simulink model "xEMU_SimulationModel3_rule1"  (R2017b)
settings: Solver=ode4  StartTime=0.0  StopTime=8192  FixedStep=0.01  RelTol=1e-3
undefined symbols (not defined in the file): a1, a2, a3, a4, ACO, BAT, Battery, DCT, DRT, EMS, ENV, Fahrzyklus_VS_modell, height_BAT, leistung, lib_bat, Maximum, Maximum_position, Num_cells, P_FC_max_long, P_FC_min_long, P_FC_step_max, Pbat_charge_max, Pbat_discharge_max, Pfc_max, Pfc_min, SOC_tar, time_peaks, TRM, velocity_peaks
libraries: simulink x5
(part 11 of 15)

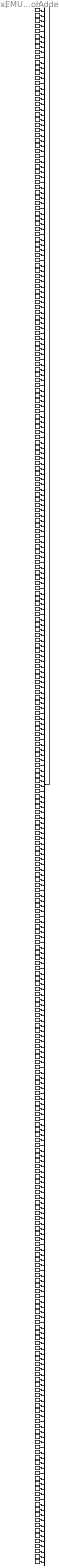
== system xEMU_SimulationModel3_rule1/Battery (BAT)_komplex/Subsystem/Thermal/Coolings/CoolAdder ==
  P_cool : Inport
  Add_FV_{1..300} (300 alike) : Sum  Inputs=-
  Demux : Demux  Outputs=2
  Mux : Mux  Inputs=300
  P_FV : Outport
  wires:
  P_cool/1 -> Demux/1
  Mux/1 -> P_FV/1
  Add_FV_1/1 -> Mux/1
  Add_FV_2/1 -> Mux/2
  Add_FV_3/1 -> Mux/3
  Add_FV_4/1 -> Mux/4
  Add_FV_5/1 -> Mux/5
  Add_FV_6/1 -> Mux/6
  Add_FV_7/1 -> Mux/7
  Add_FV_8/1 -> Mux/8
  Add_FV_9/1 -> Mux/9
  Add_FV_10/1 -> Mux/10
  Add_FV_11/1 -> Mux/11
  Add_FV_12/1 -> Mux/12
  Add_FV_13/1 -> Mux/13
  Add_FV_14/1 -> Mux/14
  Add_FV_15/1 -> Mux/15
  Add_FV_16/1 -> Mux/16
  Add_FV_17/1 -> Mux/17
  Add_FV_18/1 -> Mux/18
  Add_FV_19/1 -> Mux/19
  Add_FV_20/1 -> Mux/20
  Add_FV_21/1 -> Mux/21
  Add_FV_22/1 -> Mux/22
  Add_FV_23/1 -> Mux/23
  Add_FV_24/1 -> Mux/24
  Add_FV_25/1 -> Mux/25
  Add_FV_26/1 -> Mux/26
  Add_FV_27/1 -> Mux/27
  Add_FV_28/1 -> Mux/28
  Add_FV_29/1 -> Mux/29
  Add_FV_30/1 -> Mux/30
  Add_FV_31/1 -> Mux/31
  Add_FV_32/1 -> Mux/32
  Add_FV_33/1 -> Mux/33
  Add_FV_34/1 -> Mux/34
  Add_FV_35/1 -> Mux/35
  Add_FV_36/1 -> Mux/36
  Add_FV_37/1 -> Mux/37
  Add_FV_38/1 -> Mux/38
  Add_FV_39/1 -> Mux/39
  Add_FV_40/1 -> Mux/40
  Add_FV_41/1 -> Mux/41
  Add_FV_42/1 -> Mux/42
  Add_FV_43/1 -> Mux/43
  Add_FV_44/1 -> Mux/44
  Add_FV_45/1 -> Mux/45
  Add_FV_46/1 -> Mux/46
  Add_FV_47/1 -> Mux/47
  Add_FV_48/1 -> Mux/48
  Add_FV_49/1 -> Mux/49
  Add_FV_50/1 -> Mux/50
  Add_FV_51/1 -> Mux/51
  Add_FV_52/1 -> Mux/52
  Add_FV_53/1 -> Mux/53
  Add_FV_54/1 -> Mux/54
  Add_FV_55/1 -> Mux/55
  Add_FV_56/1 -> Mux/56
  Add_FV_57/1 -> Mux/57
  Add_FV_58/1 -> Mux/58
  Add_FV_59/1 -> Mux/59
  Add_FV_60/1 -> Mux/60
  Add_FV_61/1 -> Mux/61
  Add_FV_62/1 -> Mux/62
  Add_FV_63/1 -> Mux/63
  Add_FV_64/1 -> Mux/64
  Add_FV_65/1 -> Mux/65
  Add_FV_66/1 -> Mux/66
  Add_FV_67/1 -> Mux/67
  Add_FV_68/1 -> Mux/68
  Add_FV_69/1 -> Mux/69
  Add_FV_70/1 -> Mux/70
  Add_FV_71/1 -> Mux/71
  Add_FV_72/1 -> Mux/72
  Add_FV_73/1 -> Mux/73
  Add_FV_74/1 -> Mux/74
  Add_FV_75/1 -> Mux/75
  Add_FV_76/1 -> Mux/76
  Add_FV_77/1 -> Mux/77
  Add_FV_78/1 -> Mux/78
  Add_FV_79/1 -> Mux/79
  Add_FV_80/1 -> Mux/80
  Add_FV_81/1 -> Mux/81
  Add_FV_82/1 -> Mux/82
  Add_FV_83/1 -> Mux/83
  Add_FV_84/1 -> Mux/84
  Add_FV_85/1 -> Mux/85
  Add_FV_86/1 -> Mux/86
  Add_FV_87/1 -> Mux/87
  Add_FV_88/1 -> Mux/88
  Add_FV_89/1 -> Mux/89
  Add_FV_90/1 -> Mux/90
  Add_FV_91/1 -> Mux/91
  Add_FV_92/1 -> Mux/92
  Add_FV_93/1 -> Mux/93
  Add_FV_94/1 -> Mux/94
  Add_FV_95/1 -> Mux/95
  Add_FV_96/1 -> Mux/96
  Add_FV_97/1 -> Mux/97
  Add_FV_98/1 -> Mux/98
  Add_FV_99/1 -> Mux/99
  Add_FV_100/1 -> Mux/100
  Add_FV_101/1 -> Mux/101
  Add_FV_102/1 -> Mux/102
  Add_FV_103/1 -> Mux/103
  Add_FV_104/1 -> Mux/104
  Add_FV_105/1 -> Mux/105
  Add_FV_106/1 -> Mux/106
  Add_FV_107/1 -> Mux/107
  Add_FV_108/1 -> Mux/108
  Add_FV_109/1 -> Mux/109
  Add_FV_110/1 -> Mux/110
  Add_FV_111/1 -> Mux/111
  Add_FV_112/1 -> Mux/112
  Add_FV_113/1 -> Mux/113
  Add_FV_114/1 -> Mux/114
  Add_FV_115/1 -> Mux/115
  Add_FV_116/1 -> Mux/116
  Add_FV_117/1 -> Mux/117
  Add_FV_118/1 -> Mux/118
  Add_FV_119/1 -> Mux/119
  Add_FV_120/1 -> Mux/120
  Add_FV_121/1 -> Mux/121
  Add_FV_122/1 -> Mux/122
  Add_FV_123/1 -> Mux/123
  Add_FV_124/1 -> Mux/124
  Add_FV_125/1 -> Mux/125
  Add_FV_126/1 -> Mux/126
  Add_FV_127/1 -> Mux/127
  Add_FV_128/1 -> Mux/128
  Add_FV_129/1 -> Mux/129
  Add_FV_130/1 -> Mux/130
  Add_FV_131/1 -> Mux/131
  Add_FV_132/1 -> Mux/132
  Add_FV_133/1 -> Mux/133
  Add_FV_134/1 -> Mux/134
  Add_FV_135/1 -> Mux/135
  Add_FV_136/1 -> Mux/136
  Add_FV_137/1 -> Mux/137
  Add_FV_138/1 -> Mux/138
  Add_FV_139/1 -> Mux/139
  Add_FV_140/1 -> Mux/140
  Add_FV_141/1 -> Mux/141
  Add_FV_142/1 -> Mux/142
  Add_FV_143/1 -> Mux/143
  Add_FV_144/1 -> Mux/144
  Add_FV_145/1 -> Mux/145
  Add_FV_146/1 -> Mux/146
  Add_FV_147/1 -> Mux/147
  Add_FV_148/1 -> Mux/148
  Add_FV_149/1 -> Mux/149
  Add_FV_150/1 -> Mux/150
  Add_FV_151/1 -> Mux/151
  Add_FV_152/1 -> Mux/152
  Add_FV_153/1 -> Mux/153
  Add_FV_154/1 -> Mux/154
  Add_FV_155/1 -> Mux/155
  Add_FV_156/1 -> Mux/156
  Add_FV_157/1 -> Mux/157
  Add_FV_158/1 -> Mux/158
  Add_FV_159/1 -> Mux/159
  Add_FV_160/1 -> Mux/160
  Add_FV_161/1 -> Mux/161
  Add_FV_162/1 -> Mux/162
  Add_FV_163/1 -> Mux/163
  Add_FV_164/1 -> Mux/164
  Add_FV_165/1 -> Mux/165
  Add_FV_166/1 -> Mux/166
  Add_FV_167/1 -> Mux/167
  Add_FV_168/1 -> Mux/168
  Add_FV_169/1 -> Mux/169
  Add_FV_170/1 -> Mux/170
  Add_FV_171/1 -> Mux/171
  Add_FV_172/1 -> Mux/172
  Add_FV_173/1 -> Mux/173
  Add_FV_174/1 -> Mux/174
  Add_FV_175/1 -> Mux/175
  Add_FV_176/1 -> Mux/176
  Add_FV_177/1 -> Mux/177
  Add_FV_178/1 -> Mux/178
  Add_FV_179/1 -> Mux/179
  Add_FV_180/1 -> Mux/180
  Add_FV_181/1 -> Mux/181
  Add_FV_182/1 -> Mux/182
  Add_FV_183/1 -> Mux/183
  Add_FV_184/1 -> Mux/184
  Add_FV_185/1 -> Mux/185
  Add_FV_186/1 -> Mux/186
  Add_FV_187/1 -> Mux/187
  Add_FV_188/1 -> Mux/188
  Add_FV_189/1 -> Mux/189
  Add_FV_190/1 -> Mux/190
  Add_FV_191/1 -> Mux/191
  Add_FV_192/1 -> Mux/192
  Add_FV_193/1 -> Mux/193
  Add_FV_194/1 -> Mux/194
  Add_FV_195/1 -> Mux/195
  Add_FV_196/1 -> Mux/196
  Add_FV_197/1 -> Mux/197
  Add_FV_198/1 -> Mux/198
  Add_FV_199/1 -> Mux/199
  Add_FV_200/1 -> Mux/200
  Add_FV_201/1 -> Mux/201
  Add_FV_202/1 -> Mux/202
  Add_FV_203/1 -> Mux/203
  Add_FV_204/1 -> Mux/204
  Add_FV_205/1 -> Mux/205
  Add_FV_206/1 -> Mux/206
  Add_FV_207/1 -> Mux/207
  Add_FV_208/1 -> Mux/208
  Add_FV_209/1 -> Mux/209
  Add_FV_210/1 -> Mux/210
  Add_FV_211/1 -> Mux/211
  Add_FV_212/1 -> Mux/212
  Add_FV_213/1 -> Mux/213
  Add_FV_214/1 -> Mux/214
  Add_FV_215/1 -> Mux/215
  Add_FV_216/1 -> Mux/216
  Add_FV_217/1 -> Mux/217
  Add_FV_218/1 -> Mux/218
  Add_FV_219/1 -> Mux/219
  Add_FV_220/1 -> Mux/220
  Add_FV_221/1 -> Mux/221
  Add_FV_222/1 -> Mux/222
  Add_FV_223/1 -> Mux/223
  Add_FV_224/1 -> Mux/224
  Add_FV_225/1 -> Mux/225
  Add_FV_226/1 -> Mux/226
  Add_FV_227/1 -> Mux/227
  Add_FV_228/1 -> Mux/228
  Add_FV_229/1 -> Mux/229
  Add_FV_230/1 -> Mux/230
  Add_FV_231/1 -> Mux/231
  Add_FV_232/1 -> Mux/232
  Add_FV_233/1 -> Mux/233
  Add_FV_234/1 -> Mux/234
  Add_FV_235/1 -> Mux/235
  Add_FV_236/1 -> Mux/236
  Add_FV_237/1 -> Mux/237
  Add_FV_238/1 -> Mux/238
  Add_FV_239/1 -> Mux/239
  Add_FV_240/1 -> Mux/240
  Add_FV_241/1 -> Mux/241
  Add_FV_242/1 -> Mux/242
  Add_FV_243/1 -> Mux/243
  Add_FV_244/1 -> Mux/244
  Add_FV_245/1 -> Mux/245
  Add_FV_246/1 -> Mux/246
  Add_FV_247/1 -> Mux/247
  Add_FV_248/1 -> Mux/248
  Add_FV_249/1 -> Mux/249
  Add_FV_250/1 -> Mux/250
  Add_FV_251/1 -> Mux/251
  Add_FV_252/1 -> Mux/252
  Add_FV_253/1 -> Mux/253
  Add_FV_254/1 -> Mux/254
  Add_FV_255/1 -> Mux/255
  Add_FV_256/1 -> Mux/256
  Add_FV_257/1 -> Mux/257
  Add_FV_258/1 -> Mux/258
  Add_FV_259/1 -> Mux/259
  Add_FV_260/1 -> Mux/260
  Add_FV_261/1 -> Mux/261
  Add_FV_262/1 -> Mux/262
  Add_FV_263/1 -> Mux/263
  Add_FV_264/1 -> Mux/264
  Add_FV_265/1 -> Mux/265
  Add_FV_266/1 -> Mux/266
  Add_FV_267/1 -> Mux/267
  Add_FV_268/1 -> Mux/268
  Add_FV_269/1 -> Mux/269
  Add_FV_270/1 -> Mux/270
  Add_FV_271/1 -> Mux/271
  Add_FV_272/1 -> Mux/272
  Add_FV_273/1 -> Mux/273
  Add_FV_274/1 -> Mux/274
  Add_FV_275/1 -> Mux/275
  Add_FV_276/1 -> Mux/276
  Add_FV_277/1 -> Mux/277
  Add_FV_278/1 -> Mux/278
  Add_FV_279/1 -> Mux/279
  Add_FV_280/1 -> Mux/280
  Add_FV_281/1 -> Mux/281
  Add_FV_282/1 -> Mux/282
  Add_FV_283/1 -> Mux/283
  Add_FV_284/1 -> Mux/284
  Add_FV_285/1 -> Mux/285
  Add_FV_286/1 -> Mux/286
  Add_FV_287/1 -> Mux/287
  Add_FV_288/1 -> Mux/288
  Add_FV_289/1 -> Mux/289
  Add_FV_290/1 -> Mux/290
  Add_FV_291/1 -> Mux/291
  Add_FV_292/1 -> Mux/292
  Add_FV_293/1 -> Mux/293
  Add_FV_294/1 -> Mux/294
  Add_FV_295/1 -> Mux/295
  Add_FV_296/1 -> Mux/296
  Add_FV_297/1 -> Mux/297
  Add_FV_298/1 -> Mux/298
  Add_FV_299/1 -> Mux/299
  Add_FV_300/1 -> Mux/300

== system xEMU_SimulationModel3_rule1/Battery (BAT)_mittel/Battery/ElectricalCircuit/SerialTwoPort_Elem1/Cellelement_Elem1 ==
  OhmicResistance_Elem4 : Subsystem
  ParallelRC_Elem1 : Subsystem
  ParallelRC_Elem2 : Subsystem
  ParallelRC_Elem3 : Subsystem
  SoC : Integrator  InitialCondition=SOC_tar*100  LimitOutput=on  UpperSaturationLimit=100  LowerSaturationLimit=0
  SoCFactor : Gain  Gain=0.0012077
  VoltageSource_Elem5 : Subsystem
  tag scope: SoC1=scoped
  wires:
  [I_CellElement1] -> SoCFactor/1
  SoCFactor/1 -> SoC/1
  SoC/1 -> OhmicResistance_Elem4/2(SoC), VoltageSource_Elem5/2(SoC), ParallelRC_Elem3/2(SoC), ParallelRC_Elem2/2(SoC), ParallelRC_Elem1/2(SoC), [SoC1]
  [T_CellElement1] -> OhmicResistance_Elem4/1(T), VoltageSource_Elem5/1(T), ParallelRC_Elem3/1(T), ParallelRC_Elem2/1(T), ParallelRC_Elem1/1(T)

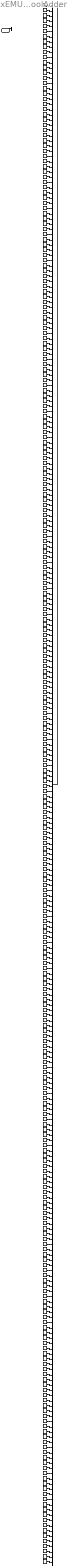
== system xEMU_SimulationModel3_rule1/Battery (BAT)_mittel/Battery/Thermal/Coolings/CoolAdder ==
  P_cool : Inport
  Add_FV_{1..300} (300 alike) : Sum  Inputs=-
  Demux : Demux  Outputs=2
  Mux : Mux  Inputs=300
  P_FV : Outport
  wires:
  P_cool/1 -> Demux/1
  Mux/1 -> P_FV/1
  Add_FV_1/1 -> Mux/1
  Add_FV_2/1 -> Mux/2
  Add_FV_3/1 -> Mux/3
  Add_FV_4/1 -> Mux/4
  Add_FV_5/1 -> Mux/5
  Add_FV_6/1 -> Mux/6
  Add_FV_7/1 -> Mux/7
  Add_FV_8/1 -> Mux/8
  Add_FV_9/1 -> Mux/9
  Add_FV_10/1 -> Mux/10
  Add_FV_11/1 -> Mux/11
  Add_FV_12/1 -> Mux/12
  Add_FV_13/1 -> Mux/13
  Add_FV_14/1 -> Mux/14
  Add_FV_15/1 -> Mux/15
  Add_FV_16/1 -> Mux/16
  Add_FV_17/1 -> Mux/17
  Add_FV_18/1 -> Mux/18
  Add_FV_19/1 -> Mux/19
  Add_FV_20/1 -> Mux/20
  Add_FV_21/1 -> Mux/21
  Add_FV_22/1 -> Mux/22
  Add_FV_23/1 -> Mux/23
  Add_FV_24/1 -> Mux/24
  Add_FV_25/1 -> Mux/25
  Add_FV_26/1 -> Mux/26
  Add_FV_27/1 -> Mux/27
  Add_FV_28/1 -> Mux/28
  Add_FV_29/1 -> Mux/29
  Add_FV_30/1 -> Mux/30
  Add_FV_31/1 -> Mux/31
  Add_FV_32/1 -> Mux/32
  Add_FV_33/1 -> Mux/33
  Add_FV_34/1 -> Mux/34
  Add_FV_35/1 -> Mux/35
  Add_FV_36/1 -> Mux/36
  Add_FV_37/1 -> Mux/37
  Add_FV_38/1 -> Mux/38
  Add_FV_39/1 -> Mux/39
  Add_FV_40/1 -> Mux/40
  Add_FV_41/1 -> Mux/41
  Add_FV_42/1 -> Mux/42
  Add_FV_43/1 -> Mux/43
  Add_FV_44/1 -> Mux/44
  Add_FV_45/1 -> Mux/45
  Add_FV_46/1 -> Mux/46
  Add_FV_47/1 -> Mux/47
  Add_FV_48/1 -> Mux/48
  Add_FV_49/1 -> Mux/49
  Add_FV_50/1 -> Mux/50
  Add_FV_51/1 -> Mux/51
  Add_FV_52/1 -> Mux/52
  Add_FV_53/1 -> Mux/53
  Add_FV_54/1 -> Mux/54
  Add_FV_55/1 -> Mux/55
  Add_FV_56/1 -> Mux/56
  Add_FV_57/1 -> Mux/57
  Add_FV_58/1 -> Mux/58
  Add_FV_59/1 -> Mux/59
  Add_FV_60/1 -> Mux/60
  Add_FV_61/1 -> Mux/61
  Add_FV_62/1 -> Mux/62
  Add_FV_63/1 -> Mux/63
  Add_FV_64/1 -> Mux/64
  Add_FV_65/1 -> Mux/65
  Add_FV_66/1 -> Mux/66
  Add_FV_67/1 -> Mux/67
  Add_FV_68/1 -> Mux/68
  Add_FV_69/1 -> Mux/69
  Add_FV_70/1 -> Mux/70
  Add_FV_71/1 -> Mux/71
  Add_FV_72/1 -> Mux/72
  Add_FV_73/1 -> Mux/73
  Add_FV_74/1 -> Mux/74
  Add_FV_75/1 -> Mux/75
  Add_FV_76/1 -> Mux/76
  Add_FV_77/1 -> Mux/77
  Add_FV_78/1 -> Mux/78
  Add_FV_79/1 -> Mux/79
  Add_FV_80/1 -> Mux/80
  Add_FV_81/1 -> Mux/81
  Add_FV_82/1 -> Mux/82
  Add_FV_83/1 -> Mux/83
  Add_FV_84/1 -> Mux/84
  Add_FV_85/1 -> Mux/85
  Add_FV_86/1 -> Mux/86
  Add_FV_87/1 -> Mux/87
  Add_FV_88/1 -> Mux/88
  Add_FV_89/1 -> Mux/89
  Add_FV_90/1 -> Mux/90
  Add_FV_91/1 -> Mux/91
  Add_FV_92/1 -> Mux/92
  Add_FV_93/1 -> Mux/93
  Add_FV_94/1 -> Mux/94
  Add_FV_95/1 -> Mux/95
  Add_FV_96/1 -> Mux/96
  Add_FV_97/1 -> Mux/97
  Add_FV_98/1 -> Mux/98
  Add_FV_99/1 -> Mux/99
  Add_FV_100/1 -> Mux/100
  Add_FV_101/1 -> Mux/101
  Add_FV_102/1 -> Mux/102
  Add_FV_103/1 -> Mux/103
  Add_FV_104/1 -> Mux/104
  Add_FV_105/1 -> Mux/105
  Add_FV_106/1 -> Mux/106
  Add_FV_107/1 -> Mux/107
  Add_FV_108/1 -> Mux/108
  Add_FV_109/1 -> Mux/109
  Add_FV_110/1 -> Mux/110
  Add_FV_111/1 -> Mux/111
  Add_FV_112/1 -> Mux/112
  Add_FV_113/1 -> Mux/113
  Add_FV_114/1 -> Mux/114
  Add_FV_115/1 -> Mux/115
  Add_FV_116/1 -> Mux/116
  Add_FV_117/1 -> Mux/117
  Add_FV_118/1 -> Mux/118
  Add_FV_119/1 -> Mux/119
  Add_FV_120/1 -> Mux/120
  Add_FV_121/1 -> Mux/121
  Add_FV_122/1 -> Mux/122
  Add_FV_123/1 -> Mux/123
  Add_FV_124/1 -> Mux/124
  Add_FV_125/1 -> Mux/125
  Add_FV_126/1 -> Mux/126
  Add_FV_127/1 -> Mux/127
  Add_FV_128/1 -> Mux/128
  Add_FV_129/1 -> Mux/129
  Add_FV_130/1 -> Mux/130
  Add_FV_131/1 -> Mux/131
  Add_FV_132/1 -> Mux/132
  Add_FV_133/1 -> Mux/133
  Add_FV_134/1 -> Mux/134
  Add_FV_135/1 -> Mux/135
  Add_FV_136/1 -> Mux/136
  Add_FV_137/1 -> Mux/137
  Add_FV_138/1 -> Mux/138
  Add_FV_139/1 -> Mux/139
  Add_FV_140/1 -> Mux/140
  Add_FV_141/1 -> Mux/141
  Add_FV_142/1 -> Mux/142
  Add_FV_143/1 -> Mux/143
  Add_FV_144/1 -> Mux/144
  Add_FV_145/1 -> Mux/145
  Add_FV_146/1 -> Mux/146
  Add_FV_147/1 -> Mux/147
  Add_FV_148/1 -> Mux/148
  Add_FV_149/1 -> Mux/149
  Add_FV_150/1 -> Mux/150
  Add_FV_151/1 -> Mux/151
  Add_FV_152/1 -> Mux/152
  Add_FV_153/1 -> Mux/153
  Add_FV_154/1 -> Mux/154
  Add_FV_155/1 -> Mux/155
  Add_FV_156/1 -> Mux/156
  Add_FV_157/1 -> Mux/157
  Add_FV_158/1 -> Mux/158
  Add_FV_159/1 -> Mux/159
  Add_FV_160/1 -> Mux/160
  Add_FV_161/1 -> Mux/161
  Add_FV_162/1 -> Mux/162
  Add_FV_163/1 -> Mux/163
  Add_FV_164/1 -> Mux/164
  Add_FV_165/1 -> Mux/165
  Add_FV_166/1 -> Mux/166
  Add_FV_167/1 -> Mux/167
  Add_FV_168/1 -> Mux/168
  Add_FV_169/1 -> Mux/169
  Add_FV_170/1 -> Mux/170
  Add_FV_171/1 -> Mux/171
  Add_FV_172/1 -> Mux/172
  Add_FV_173/1 -> Mux/173
  Add_FV_174/1 -> Mux/174
  Add_FV_175/1 -> Mux/175
  Add_FV_176/1 -> Mux/176
  Add_FV_177/1 -> Mux/177
  Add_FV_178/1 -> Mux/178
  Add_FV_179/1 -> Mux/179
  Add_FV_180/1 -> Mux/180
  Add_FV_181/1 -> Mux/181
  Add_FV_182/1 -> Mux/182
  Add_FV_183/1 -> Mux/183
  Add_FV_184/1 -> Mux/184
  Add_FV_185/1 -> Mux/185
  Add_FV_186/1 -> Mux/186
  Add_FV_187/1 -> Mux/187
  Add_FV_188/1 -> Mux/188
  Add_FV_189/1 -> Mux/189
  Add_FV_190/1 -> Mux/190
  Add_FV_191/1 -> Mux/191
  Add_FV_192/1 -> Mux/192
  Add_FV_193/1 -> Mux/193
  Add_FV_194/1 -> Mux/194
  Add_FV_195/1 -> Mux/195
  Add_FV_196/1 -> Mux/196
  Add_FV_197/1 -> Mux/197
  Add_FV_198/1 -> Mux/198
  Add_FV_199/1 -> Mux/199
  Add_FV_200/1 -> Mux/200
  Add_FV_201/1 -> Mux/201
  Add_FV_202/1 -> Mux/202
  Add_FV_203/1 -> Mux/203
  Add_FV_204/1 -> Mux/204
  Add_FV_205/1 -> Mux/205
  Add_FV_206/1 -> Mux/206
  Add_FV_207/1 -> Mux/207
  Add_FV_208/1 -> Mux/208
  Add_FV_209/1 -> Mux/209
  Add_FV_210/1 -> Mux/210
  Add_FV_211/1 -> Mux/211
  Add_FV_212/1 -> Mux/212
  Add_FV_213/1 -> Mux/213
  Add_FV_214/1 -> Mux/214
  Add_FV_215/1 -> Mux/215
  Add_FV_216/1 -> Mux/216
  Add_FV_217/1 -> Mux/217
  Add_FV_218/1 -> Mux/218
  Add_FV_219/1 -> Mux/219
  Add_FV_220/1 -> Mux/220
  Add_FV_221/1 -> Mux/221
  Add_FV_222/1 -> Mux/222
  Add_FV_223/1 -> Mux/223
  Add_FV_224/1 -> Mux/224
  Add_FV_225/1 -> Mux/225
  Add_FV_226/1 -> Mux/226
  Add_FV_227/1 -> Mux/227
  Add_FV_228/1 -> Mux/228
  Add_FV_229/1 -> Mux/229
  Add_FV_230/1 -> Mux/230
  Add_FV_231/1 -> Mux/231
  Add_FV_232/1 -> Mux/232
  Add_FV_233/1 -> Mux/233
  Add_FV_234/1 -> Mux/234
  Add_FV_235/1 -> Mux/235
  Add_FV_236/1 -> Mux/236
  Add_FV_237/1 -> Mux/237
  Add_FV_238/1 -> Mux/238
  Add_FV_239/1 -> Mux/239
  Add_FV_240/1 -> Mux/240
  Add_FV_241/1 -> Mux/241
  Add_FV_242/1 -> Mux/242
  Add_FV_243/1 -> Mux/243
  Add_FV_244/1 -> Mux/244
  Add_FV_245/1 -> Mux/245
  Add_FV_246/1 -> Mux/246
  Add_FV_247/1 -> Mux/247
  Add_FV_248/1 -> Mux/248
  Add_FV_249/1 -> Mux/249
  Add_FV_250/1 -> Mux/250
  Add_FV_251/1 -> Mux/251
  Add_FV_252/1 -> Mux/252
  Add_FV_253/1 -> Mux/253
  Add_FV_254/1 -> Mux/254
  Add_FV_255/1 -> Mux/255
  Add_FV_256/1 -> Mux/256
  Add_FV_257/1 -> Mux/257
  Add_FV_258/1 -> Mux/258
  Add_FV_259/1 -> Mux/259
  Add_FV_260/1 -> Mux/260
  Add_FV_261/1 -> Mux/261
  Add_FV_262/1 -> Mux/262
  Add_FV_263/1 -> Mux/263
  Add_FV_264/1 -> Mux/264
  Add_FV_265/1 -> Mux/265
  Add_FV_266/1 -> Mux/266
  Add_FV_267/1 -> Mux/267
  Add_FV_268/1 -> Mux/268
  Add_FV_269/1 -> Mux/269
  Add_FV_270/1 -> Mux/270
  Add_FV_271/1 -> Mux/271
  Add_FV_272/1 -> Mux/272
  Add_FV_273/1 -> Mux/273
  Add_FV_274/1 -> Mux/274
  Add_FV_275/1 -> Mux/275
  Add_FV_276/1 -> Mux/276
  Add_FV_277/1 -> Mux/277
  Add_FV_278/1 -> Mux/278
  Add_FV_279/1 -> Mux/279
  Add_FV_280/1 -> Mux/280
  Add_FV_281/1 -> Mux/281
  Add_FV_282/1 -> Mux/282
  Add_FV_283/1 -> Mux/283
  Add_FV_284/1 -> Mux/284
  Add_FV_285/1 -> Mux/285
  Add_FV_286/1 -> Mux/286
  Add_FV_287/1 -> Mux/287
  Add_FV_288/1 -> Mux/288
  Add_FV_289/1 -> Mux/289
  Add_FV_290/1 -> Mux/290
  Add_FV_291/1 -> Mux/291
  Add_FV_292/1 -> Mux/292
  Add_FV_293/1 -> Mux/293
  Add_FV_294/1 -> Mux/294
  Add_FV_295/1 -> Mux/295
  Add_FV_296/1 -> Mux/296
  Add_FV_297/1 -> Mux/297
  Add_FV_298/1 -> Mux/298
  Add_FV_299/1 -> Mux/299
  Add_FV_300/1 -> Mux/300

== system xEMU_SimulationModel3_rule1/Battery (BAT)_mittel/Subsystem1/ElectricalCircuit/Cellelement_Elem1/OhmicResistance_Elem1 ==
  T : Inport
  SoC : Inport  Port=2
  Object : Lookup_n-D  BreakpointsForDimension1=[10 25 35 45]  BreakpointsForDimension2=[0 5 10 15 20 25 30 35 40 45 50 55 60 65 70 75 80 85 90 95 100]  Table=[0.000771968526803023 0.000748369146052688 0.000724881421092217 0.000703132225685812 0.000681405509074902 0.000662730818510104 0.000645251487485153 0.000631118585145968 0.000617074401605558 0.000603444604710944 0.000588975057934144 0.000574938504017678 0.000557784934803898 0.00054413410139131 0.0005282009160006 0.000513150140111006 0.000497368589356565 0.000480432670706108 0.000468327505260267 0.000459151981966271 0.00044721979103073;0.000607538709252138 0.000591906678896865 0.000579251526535265 0.000566736941111578 0.000554267843362006 0.00054193499054528 0.000528289326909059 0.000518627966086254 0.000508454014080012 0.000498619432440266 0.000487314814733121 0.000479311632434861 0.000469030628019127 0.000460272639433147 0.000450192255124041 0.000439297274666459 0.000428239996856566 0.000417728515462718 0.000409674349230244 0.000404459083809335 0.000392103511229194;0.000532360065388155 0.00052360448028229 0.000514747341431657 0.000504947167518555 0.00049503906759317 0.000486377259235303 0.000477750186118738 0.000468937804866539 0.000461447107731537 0.000454666596698088 0.000447908076851307 0.000441183098574019 0.000431588050586221 0.000424993386722809 0.000419393984065282 0.000411618970605753 0.000403616676362054 0.000395831770376174 0.000387955856358833 0.000382048896042462 0.000377611755738171;0.000491068260475341 0.00048241524334078 0.000478893043251579 0.000474231745067159 0.000463419524146351 0.000453533482441388 0.000448154117766324 0.000444198582958616 0.000440406492727549 0.000434596688885989 0.000428993938540256 0.000423688723613095 0.000417260659200824 0.000411063362411327 0.000403315228447255 0.00040014675568242 0.000393272441695337 0.00038814268028836 0.00038290705375794 0.000373250570942629 0.000364317930560238]  ExtrapMethod=Clip  RndMeth=Simplest  InputSameDT=on
  tag scope: ID1_ObjR=global
  wires:
  Object/1 -> [ID1_ObjR]
  T/1 -> Object/1
  SoC/1 -> Object/2

== system xEMU_SimulationModel3_rule1/Battery (BAT)_mittel/Subsystem1/ElectricalCircuit/Cellelement_Elem1/ParallelRC_Elem5 ==
  T : Inport
  SoC : Inport  Port=2
  Object : Lookup_n-D  BreakpointsForDimension1=[10 25 35 45]  BreakpointsForDimension2=[0 5 10 15 20 25 30 35 40 45 50 55 60 65 70 75 80 85 90 95 100]  Table=[0.00764728927709652 0.00474423865923742 0.00203396840695321 0.00231038728921286 0.00206615832855233 0.00190458593231064 0.00185856156152465 0.00165198805708657 0.00171477833745534 0.00153065139517468 0.00163818950613008 0.00153651551312183 0.000909011357916661 0.00118776928802931 0.00170773809968292 0.00152798511163003 0.00132357118315589 0.00119016648121892 0.000863319393777177 0.0011826590260031 0.00118270083620402;0.00587553867538804 0.00154839875781604 0.00145455635275654 0.00108066337379952 0.00123647187367758 0.00134505637092348 0.00119010790610603 0.000914840836507952 0.00120902316731515 0.00106177386040427 0.00113510439044689 0.00109305083615692 0.000947546726337524 0.00125215588006856 0.00102142196697215 0.000978919305729693 0.000925383538786521 0.000739308136109667 0.000689063876872616 0.000876876834715341 0.000876880431629726;0.00139386150279849 0.00145440718530885 0.00123686321307858 0.00106972733310903 0.000902712396975044 0.000963263486504002 0.000980885342233891 0.000671712100771071 0.000985515464118976 0.000801732026212843 0.000860489547883767 0.00083824337824724 0.00101406228045639 0.000968508887655047 0.000777585656833542 0.000634467307635599 0.000508360442881214 0.000537670622708236 0.000275193202810073 0.000269396711698707 0.00026940006710819;0.000860744687168582 0.00104628594847602 0.000964774286317786 0.000903956546944867 0.0008883571130244 0.000798285384222583 0.0006483394565504 0.000535561389178171 0.000508091265821407 0.00044910739208783 0.000400866304532207 0.000417700255613791 0.00064414451482694 0.000568643085179211 0.000398699574906687 0.000347961616179267 0.000331212768477187 0.000230954269983984 0.000305644439156634 0.000129027087395457 0.000128998271017311]  ExtrapMethod=Clip  RndMeth=Simplest  InputSameDT=on
  Tau : Lookup_n-D  BreakpointsForDimension1=[10 25 35 45]  BreakpointsForDimension2=[0 5 10 15 20 25 30 35 40 45 50 55 60 65 70 75 80 85 90 95 100]  Table=[22.1898909514035 26.5842152221479 31.7411994240462 47.8251884127405 47.8565404302297 47.422670108927 51.740171298322 46.2462097099599 48.3835662371059 44.7822763601721 43.1857659402676 42.4016771471478 24.3581391906999 28.5703136670354 44.416902537374 37.3094150990016 35.3769956666779 35.4705039135581 39.8139799767232 33.3061522268275 33.30599689333;22.0049861740439 25.0221638317897 37.7189952817354 22.6587659796224 37.1615499291492 37.6703675362051 36.2787721869487 22.2875536653091 33.2265829072705 32.8555058583998 30.9807312625166 32.7305073519293 25.5650300629843 32.233048150971 25.7482720766016 26.5721540946532 25.0756848266839 26.9317784085936 24.9760975672177 24.4770988013198 24.4769865270928;21.3780024298734 32.1910645264531 35.0394493423987 33.5400382823725 29.184625958329 32.1928242068211 29.675228194561 17.74604903142 27.7270396338011 28.6090915478394 28.5868733209495 31.9498489317353 27.9848660278726 23.3533871912033 21.3971772880622 21.6270074341763 21.1486235390482 19.9929459827115 7.48768361844528 20.985018857628 20.9849996151504;15.238189698917 36.0034225048109 30.755391417161 28.529975322527 26.1807246599539 26.7135294207742 18.3293756250247 14.0981192102909 12.1591957639524 11.8539599745503 10.0876535743557 9.92575052180348 15.4595077908202 10.0151490899665 8.45913947036717 8.43707343464333 12.3511967627153 7.90200149673811 13.3035597189383 9.99100957924203 9.99099938855902]  ExtrapMethod=Clip  RndMeth=Simplest  InputSameDT=on
  tag scope: ID2_ObjR=global, ID2_ObjTau=global
  wires:
  Object/1 -> [ID2_ObjR]
  T/1 -> Object/1, Tau/1
  SoC/1 -> Object/2, Tau/2
  Tau/1 -> [ID2_ObjTau]

== system xEMU_SimulationModel3_rule1/Battery (BAT)_mittel/Subsystem1/ElectricalCircuit/Cellelement_Elem1/ParallelRC_Elem6 ==
  T : Inport
  SoC : Inport  Port=2
  Object : Lookup_n-D  BreakpointsForDimension1=[10 25 35 45]  BreakpointsForDimension2=[0 5 10 15 20 25 30 35 40 45 50 55 60 65 70 75 80 85 90 95 100]  Table=[0.00612505138589157 0.00407283419232278 0.00211029694509598 0.00158426234016647 0.00154050558572137 0.00135695046447579 0.00174483106257212 0.00128267385631804 0.0015888070219515 0.00145042307444027 0.00189788894173659 0.00191806538662505 0.00252122095787405 0.00178546502838825 0.00069277294068049 0.000722858269843324 0.000687448865120982 0.000713033101262336 0.000765267477319311 0.000747209485853623 0.000747210010492783;0.0028803728228227 0.00166494478241037 0.00130679609125278 0.0014088956332448 0.00100702693562222 0.00098864172422517 0.00111459557282459 0.00102368360719172 0.000893755458255841 0.000915978165021569 0.000912913896198892 0.000927851930931685 0.0006587861100766 0.000565769571977714 0.000430224974782173 0.000596297603341754 0.000638377058612318 0.000640779681863622 0.000475648188476712 0.000644113634046433 0.000644109504448214;0.00160384570742686 0.000803193890546296 0.00117020815660094 0.000822719732794618 0.000820848778809978 0.000745228772184654 0.000521027261974307 0.000675990896562611 0.0006374826532219 0.000809498752713429 0.00075344471045016 0.000777186513743439 0.000583235753089049 0.000461271319101388 0.000264239208753733 0.000315200624621732 0.000385153057603513 0.000355119347985819 0.000466231518822687 0.000385143980736301 0.000385139918760484;0.0011058837581201 0.00102327958142904 0.000854017589770261 0.000620354722485578 0.000533612297837053 0.000554932892670066 0.000545949328641521 0.000564765991762031 0.000557954507833749 0.000571334206155164 0.000611361350603188 0.000581992936132193 0.00032553522338182 0.000308453864003534 0.000245402536897638 0.000267237748104272 0.000271149225568223 0.000321983778533294 0.000321857571242993 0.000302892217354013 -1.93335457885538e-05]  ExtrapMethod=Clip  RndMeth=Simplest  InputSameDT=on
  Tau : Lookup_n-D  BreakpointsForDimension1=[10 25 35 45]  BreakpointsForDimension2=[0 5 10 15 20 25 30 35 40 45 50 55 60 65 70 75 80 85 90 95 100]  Table=[8894.04992458898 5583.22117357318 2395.80166283633 1222.27613662254 1292.01428487515 1131.61950126611 1623.83618664477 1094.67312849281 1491.82790066986 1278.05994799138 1511.7809635949 1129.87245676405 1286.93745584224 307.608419371418 476.725699330865 817.638115923972 835.62971341781 897.870159627786 1027.24664256503 940.219265730565 940.220014985091;1666.19698223227 1725.30031527279 1412.44748834952 2019.88206707202 1154.54617101241 1184.41979676773 1449.16341083556 1620.94357186667 1045.1208926029 1004.12263417972 914.704129892067 953.590993454473 855.556450253306 315.371820985523 764.232111251126 1212.1035795243 1203.87532778525 1113.94605881351 799.434252905741 1183.94384406215 1183.89402126425;1589.88514034659 650.112197316073 1467.02952638775 1041.69496288167 1117.68067213788 1010.25387619464 687.13401580774 1275.80911085289 922.171131504742 1156.04494477055 1056.70609053138 1154.31370451518 378.605742790933 794.666924710376 608.839146423894 734.769709561691 837.435325614985 712.905447599833 1042.2052053285 772.554093207652 772.54991646515;1621.53825009247 1313.72871612921 1200.47636507688 907.632286442718 757.517098195639 888.555824764039 1015.72794287654 1295.65572744615 1196.63571128977 1146.57640266193 1207.77397098176 1351.13029871221 1179.47682188115 795.706769335172 829.656008403581 808.642698694274 744.407212202976 855.955983164718 745.60016510757 845.668870041818 2073.68071042286]  ExtrapMethod=Clip  RndMeth=Simplest  InputSameDT=on
  tag scope: ID3_ObjR=global, ID3_ObjTau=global
  wires:
  Object/1 -> [ID3_ObjR]
  T/1 -> Object/1, Tau/1
  SoC/1 -> Object/2, Tau/2
  Tau/1 -> [ID3_ObjTau]

== system xEMU_SimulationModel3_rule1/Battery (BAT)_mittel/Subsystem1/ElectricalCircuit/Cellelement_Elem1/Rmphn_Elem2 ==
  T : Inport
  SoC : Inport  Port=2
  Object : Lookup_n-D  BreakpointsForDimension1=[10 25 35 45]  BreakpointsForDimension2=[0 5 10 15 20 25 30 35 40 45 50 55 60 65 70 75 80 85 90 95 100]  Table=[0.000268122505057072 0.00046251136129643 0.000643717837942068 0.000610386454678535 0.00045685192101357 0.000388035738603161 0.000336878735294759 0.000333375986684024 0.000321108800701806 0.000318973974892479 0.000303391249635262 0.000303204281029518 0.000297787044358361 0.000300249237624058 0.000298711247305386 0.000297350259051319 0.000301859274253576 0.000313998160496946 0.000341701603840128 0.000417691070242408 0.000417689978158318;0.105441120159789 0.00096755218954419 0.000529404764033394 0.000354619127347272 0.000284612269108788 0.000251721272272473 0.000252493664676402 0.000230094357795404 0.000207521825021393 0.000190441374899878 0.000178637719620051 0.000177529745884289 0.000175505765036172 0.000173031403485662 0.000172679629835472 0.000166312191557979 0.00017401143861351 0.000199341075567154 0.000255464654695431 0.00070692540667571 0.00353955118648807;0.00118157328513432 0.000748992447788816 0.000451818583841663 0.000290076474209044 0.000194362347991163 0.000143830566471477 9.92210097897263e-05 7.40619477978304e-05 4.40775921405744e-05 4.31116426933342e-05 4.09849161117321e-05 4.10541548999212e-05 3.8267267500746e-05 3.63092794956421e-05 4.14869060972538e-05 4.49104540893705e-05 4.59660513161652e-05 4.86952421140127e-05 4.94130500198532e-05 0.000127040319833249 0.000525588842740708;0.000669172169658894 0.000379477976380309 0.000231415435891332 0.000136838362951624 9.37210144790436e-05 0.00022453139764744 0.000261681601370784 0.000275717918924215 0.000343387485925263 0.000309569655761013 0.000327723280548032 0.000346361466696158 0.000355248627933966 0.000383511648660796 0.000762747032591511 0.000482937839790971 0.000437851512368699 0.000453348455645594 0.000469989279725756 0.000620721089927547 0.000273243452522911]  ExtrapMethod=Clip  RndMeth=Simplest  InputSameDT=on
  Tau : Lookup_n-D  BreakpointsForDimension1=[10 25 35 45]  BreakpointsForDimension2=[0 5 10 15 20 25 30 35 40 45 50 55 60 65 70 75 80 85 90 95 100]  Table=[0.000141955461410132 0.000108259964906405 7.80774844155858e-05 0.000101831536112891 0.000107975924751293 0.000108564940513868 0.000111641696811859 0.000113299614321864 0.000112465051722286 9.97340191359942e-05 0.000108640252661311 0.000108951310987874 0.000109254278947402 0.000109366925113906 0.000111301823135108 0.000118543460124368 0.000128410735701329 0.00012644454704452 0.000133838402973526 0.000136136544113434 9.82118308687161e-05;1.44148342133733e-06 1.04132356690357e-05 1.53197904992227e-05 1.58298746298682e-05 1.04100480339941e-05 4.49161696524291e-06 7.51385938203224e-07 1.19998828380278e-06 1.7484531583263e-06 2.24727945021076e-06 2.85288799447317e-06 2.3982374887958e-06 2.5543004122239e-06 2.84146194349035e-06 3.29845050624667e-06 4.36998458930454e-06 5.14859008826645e-06 5.1127506304825e-06 3.70215417911144e-06 1.08280333595243e-06 -3.40186367207846e-08;1e-07 1e-07 2.31775917823548e-07 5.9109862793901e-07 1.41930407022604e-06 2.53894683649514e-06 4.87494541206615e-06 8.66810441183524e-06 1.68823285933497e-05 1.74360926052191e-05 1.75424559454703e-05 1.6623303179158e-05 1.86276926994013e-05 1.90117503381529e-05 1.99503323044723e-05 2.10803940917103e-05 2.22552249334782e-05 2.42579904812111e-05 2.41449451303551e-05 1.01960705344891e-05 8.23637353204037e-07;1e-07 1e-07 1.00006555422865e-07 1.76638744052027e-07 1.40361049557971e-06 1.80241729343279e-06 1.14320296152634e-06 6.20353351220257e-07 3.57247497379756e-07 2.03111810542261e-07 1.41684357923681e-07 1.00689263423425e-07 1.01438254958135e-07 1.04869717402227e-07 1e-07 1e-07 1.00012811085513e-07 1.05628050575502e-07 2.21581233292744e-07 7.96773138822328e-07 2.25608914428729e-06]  ExtrapMethod=Clip  RndMeth=Simplest  InputSameDT=on
  tag scope: ID4_ObjCT=global, ID4_ObjMP=global
  wires:
  Object/1 -> [ID4_ObjCT]
  T/1 -> Object/1, Tau/1
  SoC/1 -> Object/2, Tau/2
  Tau/1 -> [ID4_ObjMP]

== system xEMU_SimulationModel3_rule1/Battery (BAT)_mittel/Subsystem1/ElectricalCircuit/Cellelement_Elem1/Rmphn_Elem3 ==
  T : Inport
  SoC : Inport  Port=2
  Object : Lookup_n-D  BreakpointsForDimension1=[10 25 35 45]  BreakpointsForDimension2=[0 5 10 15 20 25 30 35 40 45 50 55 60 65 70 75 80 85 90 95 100]  Table=[0.000268122505057072 0.00046251136129643 0.000643717837942068 0.000610386454678535 0.00045685192101357 0.000388035738603161 0.000336878735294759 0.000333375986684024 0.000321108800701806 0.000318973974892479 0.000303391249635262 0.000303204281029518 0.000297787044358361 0.000300249237624058 0.000298711247305386 0.000297350259051319 0.000301859274253576 0.000313998160496946 0.000341701603840128 0.000417691070242408 0.000417689978158318;0.105441120159789 0.00096755218954419 0.000529404764033394 0.000354619127347272 0.000284612269108788 0.000251721272272473 0.000252493664676402 0.000230094357795404 0.000207521825021393 0.000190441374899878 0.000178637719620051 0.000177529745884289 0.000175505765036172 0.000173031403485662 0.000172679629835472 0.000166312191557979 0.00017401143861351 0.000199341075567154 0.000255464654695431 0.00070692540667571 0.00353955118648807;0.00118157328513432 0.000748992447788816 0.000451818583841663 0.000290076474209044 0.000194362347991163 0.000143830566471477 9.92210097897263e-05 7.40619477978304e-05 4.40775921405744e-05 4.31116426933342e-05 4.09849161117321e-05 4.10541548999212e-05 3.8267267500746e-05 3.63092794956421e-05 4.14869060972538e-05 4.49104540893705e-05 4.59660513161652e-05 4.86952421140127e-05 4.94130500198532e-05 0.000127040319833249 0.000525588842740708;0.000669172169658894 0.000379477976380309 0.000231415435891332 0.000136838362951624 9.37210144790436e-05 0.00022453139764744 0.000261681601370784 0.000275717918924215 0.000343387485925263 0.000309569655761013 0.000327723280548032 0.000346361466696158 0.000355248627933966 0.000383511648660796 0.000762747032591511 0.000482937839790971 0.000437851512368699 0.000453348455645594 0.000469989279725756 0.000620721089927547 0.000273243452522911]  ExtrapMethod=Clip  RndMeth=Simplest  InputSameDT=on
  Tau : Lookup_n-D  BreakpointsForDimension1=[10 25 35 45]  BreakpointsForDimension2=[0 5 10 15 20 25 30 35 40 45 50 55 60 65 70 75 80 85 90 95 100]  Table=[0.000529292712630017 0.000351382846491099 0.000177810480944207 7.79403990960714e-05 6.81569541336992e-05 5.91040264946733e-05 5.28632407026636e-05 3.86685791728393e-05 3.41763608587333e-05 3.90598295370642e-05 3.33343419869487e-05 3.31788561799858e-05 3.72164662468986e-05 3.7819623059679e-05 3.92982398452099e-05 3.90459805088247e-05 3.94718130171938e-05 5.00153524126515e-05 5.77919815211187e-05 6.30552678733864e-05 0.000194648514008883;5.50411647601813e-06 3.52318210856722e-05 3.07460510072176e-05 2.88125567107061e-05 3.20934600958392e-05 3.98196491910542e-05 4.70065039136467e-05 4.16667581912915e-05 3.8766931651523e-05 3.73480760967852e-05 3.75368686771652e-05 3.79235652388832e-05 3.82366651889809e-05 3.77564206326725e-05 3.77697732369037e-05 3.92608610070005e-05 4.09722828338765e-05 4.41317395295982e-05 4.92214251960363e-05 4.91775019181766e-05 2.37762839960349e-06;2.79835750709802e-05 2.77652269593851e-05 2.59170689623705e-05 2.30145827749915e-05 2.06316035856238e-05 1.73996721774708e-05 1.69083782724042e-05 1.54723392916681e-05 1.54113892744735e-05 1.29818644067297e-05 1.18550990934711e-05 1.13907271327181e-05 1.16978907519504e-05 1.16639401630886e-05 6.99591929291379e-06 5.60005970916921e-06 6.20584876015212e-06 7.3565325766759e-06 1.5073212633788e-05 1.73520798215733e-05 1.32236073562572e-05;1.88609117562345e-05 1.56983515705563e-05 1.13522959669512e-05 8.43457227299759e-06 5.05996632935698e-06 1.95249155023466e-07 1.76960347573296e-07 1.67193948116137e-07 1.13790792161104e-07 1.54842321962181e-07 1.59787929658381e-07 1.79195596001854e-07 1.93858272726632e-07 1.959423113329e-07 1.0263240562418e-07 1.4811966509328e-07 2.15247631988995e-07 2.26942289219901e-07 2.61537981718251e-07 6.32640243600376e-07 6.94233450436108e-06]  ExtrapMethod=Clip  RndMeth=Simplest  InputSameDT=on
  tag scope: ID5_ObjCT=global, ID5_ObjMP=global
  wires:
  Object/1 -> [ID5_ObjCT]
  T/1 -> Object/1, Tau/1
  SoC/1 -> Object/2, Tau/2
  Tau/1 -> [ID5_ObjMP]

== system xEMU_SimulationModel3_rule1/Battery (BAT)_mittel/Subsystem1/ElectricalCircuit/Cellelement_Elem1/SphericalDiffusion_Elem4 ==
  T : Inport
  SoC : Inport  Port=2
  Object : Lookup_n-D  BreakpointsForDimension1=[10 25 35 45]  BreakpointsForDimension2=[0 5 10 15 20 25 30 35 40 45 50 55 60 65 70 75 80 85 90 95 100]  Table=[0.00430313409541137 0.00258316736106707 0.000909014786104972 1.18545506602962e-05 4.38366113693087e-05 8.77044399626091e-05 5.79079218847818e-05 0.000150514980577749 9.33787733777284e-05 0.000170587402323895 9.16912408369071e-05 0.000169973923190152 0.0010864171289951 0.0010168205375952 5.17594049421499e-05 5.25039764358344e-05 7.13543000736091e-05 9.72674277356414e-05 0.000262863352777946 6.70953684616619e-05 6.70949924803742e-05;0.00202864818193681 0.000693578367286168 0.000184380393678643 0.000403287595693715 0.000127662300666302 4.76087328882778e-05 0.000131120918827474 0.000337353209406746 6.4631465676567e-05 0.000123474566106843 8.04635241293952e-05 0.000162451054715727 0.000533166288895852 7.92410317103854e-05 8.48020493836965e-05 5.24883118428218e-05 2.91838096707873e-05 0.000114184116093498 0.000126907742418507 1.73539545684722e-05 1.73540061952083e-05;0.00103112903028711 4.07365124309712e-05 3.42260849887195e-05 6.30654379412048e-05 0.00016624324470566 9.00400976993266e-05 6.22392485080555e-05 0.00029158679942256 5.17588808408712e-05 0.000140058855505779 9.00232650693359e-05 8.92568237263442e-05 5.25312934291685e-05 8.92665162019484e-05 5.22566775637766e-05 0.000100524062848508 0.000141278584594374 0.000119351605629175 0.000299281628089723 0.00026149287385724 0.000261489941349852;0.000621026899352884 5.60368895320236e-05 3.18742117279188e-05 4.05885789487214e-05 3.91921275086055e-05 7.19709567229367e-05 0.000189740995702097 0.000253909950020527 0.000269517412491939 0.000277425145551863 0.000296662547586413 0.000291880241147839 0.00023830686533216 0.000175595640657073 0.000217368080740519 0.000222023403173585 0.000184231812431194 0.0002351483403811 0.000169922728749226 0.000268921139693127 0.00026891992725363]  ExtrapMethod=Clip  RndMeth=Simplest  InputSameDT=on
  Tau : Lookup_n-D  BreakpointsForDimension1=[10 25 35 45]  BreakpointsForDimension2=[0 5 10 15 20 25 30 35 40 45 50 55 60 65 70 75 80 85 90 95 100]  Table=[1115.38517775812 684.657648467646 263.177144419379 3.81744728467607 15.1293962439251 30.9953004856576 20.1374386136996 46.1976468763129 24.3342331115565 36.3078360953177 16.0981709839934 33.6491773394059 348.511561205692 928.37037442187 12.4483953448915 9.53242773674869 11.3400431038893 14.0420254456782 35.6196175844955 5.18032976962323 5.18029939245667;436.05721547597 178.788072232168 55.3194371233784 131.268654128176 44.6888118749279 17.3143772686759 44.9030974055553 105.796849607155 16.2649172847531 26.9015680841646 14.7268525811286 49.9719994898928 229.019627822504 43.8344050464637 18.918379680171 9.58535878036457 4.50330552785554 16.5919956763023 17.1024869877413 1.47841513907696 1.47839793558041;224.745225665794 10.4369473657352 10.1100156485882 20.6404452475675 59.9999171658416 33.7203018879835 22.2490337021504 92.460322726672 13.7046257706988 30.9800391075748 16.5730721535485 17.2353609039221 29.7188074063282 41.244592651443 11.3392979117728 18.0373016773353 22.5168418427195 17.3027128393532 40.2554135594826 22.7934252028777 22.7929913223903;132.312832757629 14.8466722088249 9.50749347362856 13.5149063331701 14.1435250573307 27.3268542237605 70.5271372880475 83.4077698431377 73.7985753726319 61.9682148848562 55.6945245498801 65.449708470853 159.041871284961 66.2172719242345 46.1341060367769 39.5262197327382 29.1421856819277 33.9899451331094 21.9811449727135 21.6842433004828 1.05441000209685]  ExtrapMethod=Clip  RndMeth=Simplest  InputSameDT=on
  tag scope: ID6_ObjR=global, ID6_ObjTau=global
  wires:
  Object/1 -> [ID6_ObjR]
  T/1 -> Object/1, Tau/1
  SoC/1 -> Object/2, Tau/2
  Tau/1 -> [ID6_ObjTau]
